simulink model "rtwdemo_fixpt1"  (Simulink 6.0)
settings: Solver=FixedStepDiscrete  StartTime=0.0  StopTime=1  MaxStep=.1  RelTol=1e-3
libraries: rtwdemowidgets x2
CloseFcn:
  | rtwprivate ssgencode ModelCloseRequest fpdemo
settings Model: Creator=The MathWorks Inc.  LastModifiedBy=batserve  ExtModeAutoUpdateStatusClock=off  ProdHWDeviceType=32-bit Embedded Processor
settings DataIOCC: SaveOutput=off  SaveTime=off  SignalLoggingName=sigsOut
settings OptimizationCC: InlineParams=on  EnforceIntegerDowncast=off  StateBitsets=on  DataBitsets=on  UseTempVars=on
settings DebuggingCC: CheckExecutionContextPreStartOutputMsg=on  CheckExecutionContextRuntimeOutputMsg=on  SolverPrmCheckMsg=none  ParameterOverflowMsg=warning  ParameterPrecisionLossMsg=none
settings HardwareCC: ProdHWDeviceType=32-bit Embedded Processor  TargetHWDeviceType=32-bit Generic
settings RTWCC: TLCOptions=-p0 -aWarnNonSaturatedBlocks=0  GenerateReport=on  RTWVerbose=off  ProcessScript=grt_make_rtw_hook  LaunchReport=on
settings CodeAppCC: ForceParamTrailComments=on  PrefixModelToSubsysFcnNames=off
settings GRTTargetCC: MatFileLogging=off

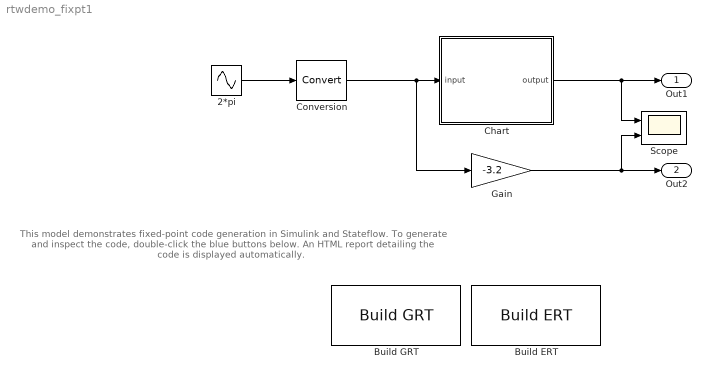
== system rtwdemo_fixpt1 ==
  note: This model demonstrates fixed-point code generation in Simulink and Stateflow.
      | To generate and inspect the code, double-click the blue buttons below.  An HTML
      | report detailing the code is displayed automatically.
  2*pi : Sin  SineType=Sample based  Frequency=2*pi  Samples=100  SampleTime=.01
  Build ERT : rtwdemowidgets/Build ERT  attrib_overrides={}
  Build GRT : rtwdemowidgets/Build GRT  attrib_overrides={}
  Chart : Stateflow chart  PropExecContextAcrossSSBoundary=on
  Conversion : DataTypeConversion  OutDataTypeMode=Specify via dialog  OutScaling=2^-4
  Gain : Gain  Gain=-3.2  ParameterDataTypeMode=Specify via dialog  ParameterScalingMode=Use specified scaling  ParameterScaling=2^-4  OutDataTypeMode=Specify via dialog  OutScaling=2^-4
  Scope : Scope  NumInputPorts=2
      settings: TimeRange=1  YMin=-2~-5  YMax=4~5
  Out1 : Outport
  Out2 : Outport  Port=2
  wires:
  2*pi/1 -> Conversion/1
  Chart/1(output) -> Out1/1, Scope/1
  Gain/1 -> Out2/1, Scope/2
  Conversion/1 -> Chart/1(input), Gain/1

== stateflow chart Chart ==
  state out = fixout(fixin) [function]
    (default) -> (junction 5)
    (junction 5) -> (junction 6) : [fixin>=0.5c]{out = 3.2c*fixin;}
    (junction 5) -> (junction 7) : {out = -3.2c*fixin;}
  (default) -> (junction 4) : {output=fixout(input);}
  data: fixin function_input fixpt size=1; out function_output fixpt size=1; input input fixpt size=1; output output fixpt size=1
